simulink model "nl_model"  (R2021b)
settings: Solver=FixedStepAuto  StartTime=0.0  StopTime=10  FixedStep=0.01  MaxStep=0.01  RelTol=1e-3
values from neighbouring files (symbols this model uses):
  circ1 = monza    [sim_data.m]
  contact_treshold = 1e2    (= 100)    [sim_data.m]
  d = 0.021    [sim_data.m]
  H_cornice = 0.005    [sim_data.m]
  ICm = [IC(2), IC(4)]    [conversion_data.m]
  Kbbx = (mb * g * rb^2 * rm) / ((mb * rb^2 + Jb) * Ly)    (= 0.952057453416)    [sim_data.m]
  Kbby = (mb * g * rb^2 * rm) / ((mb * rb^2 + Jb) * Lx)    (= 1.22502497502)    [sim_data.m]
  lm = 0.072    [sim_data.m]
  Lx = 0.143    [sim_data.m]
  Lx_cornice = 0.15    [sim_data.m]
  Lx_plane = 0.15    [sim_data.m]
  Ly = 0.184    [sim_data.m]
  Ly_cornice = 0.20    (= 0.2)    [sim_data.m]
  Ly_plane = 0.20    (= 0.2)    [sim_data.m]
  Mot_Osci_Rang = [-90 ,90]    [sim_data.m]
  pt = 0.005    [sim_data.m]
  rb = 0.02    [sim_data.m]
  rm = 0.025    [sim_data.m]
  W_cornice = 0.05    [sim_data.m]
undefined symbols (not defined in the file or in its folder): DiscIntNeverNeededParam, h, Kx, Kxi, Ky, Kyi, slow, X, Y, Z
libraries: sm_lib x75, nesl_utility x9, simulink x7, dspstat3 x5, sharedschedule x3, slpidlib x2, dspsigops x1
(part 1 of 3)
settings Model: Creator=ernesto  LastModifiedBy=ernesto

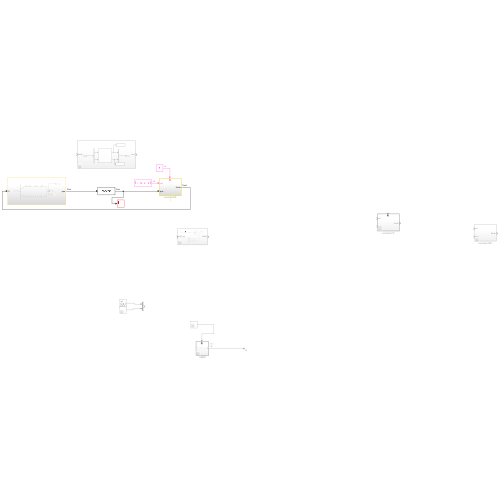
[thumbnail: Simulink's stored preview of the top-level diagram]
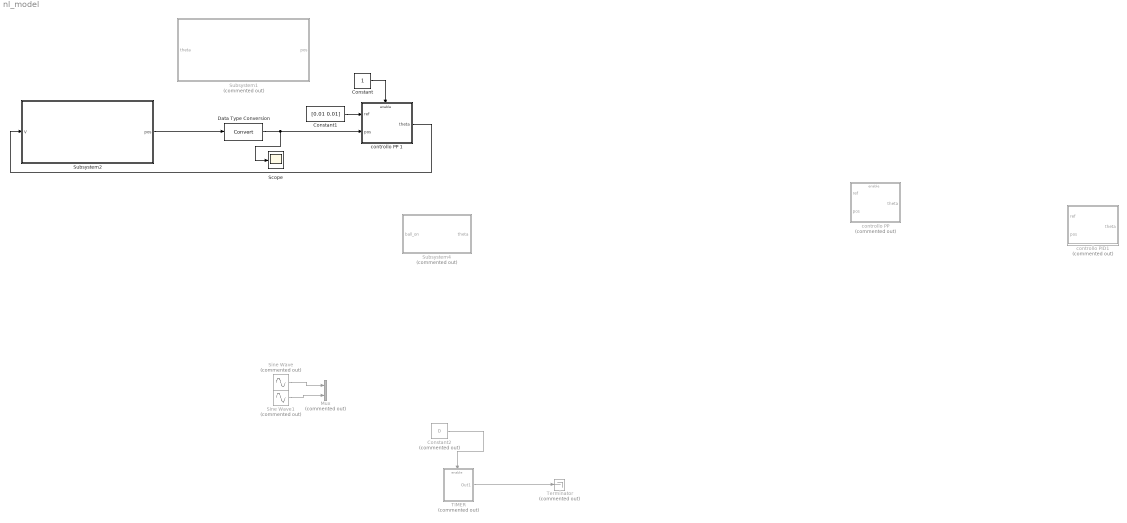
== system nl_model ==
  Constant : Constant
  Constant1 : Constant  Value=[0.01 0.01]
  Constant2 : Constant  Commented=on  Value=0  SampleTime=0.01
  Data Type Conversion : DataTypeConversion
  Mux : Mux  Commented=on  Inputs=2
  Scope : Scope
  Sine Wave : Sin  Commented=on  Amplitude=0.05  Frequency=2*pi*0.5  SampleTime=0.01
  Sine Wave1 : Sin  Commented=on  Amplitude=0.05  Frequency=2*pi*0.5  Phase=pi/2  SampleTime=0.01
  Subsystem1 : Subsystem  Commented=on
  Subsystem2 : Subsystem
  Subsystem4 : Subsystem  Commented=on
  TIMER : Subsystem  Commented=on  TreatAsAtomicUnit=on
  Terminator : Terminator  Commented=on
  controllo PID1 : Subsystem  Commented=on  SystemSampleTime=0.01
  "controllo PP " : Subsystem  Commented=on  SystemSampleTime=0.01
  controllo PP 1 : Subsystem  SystemSampleTime=0.01
  wires:
  Data Type Conversion/1 -> Scope/1, controllo PP 1/2("pos ")
  Constant2/1 -> TIMER/Enable
  TIMER/1(Out1) -> Terminator/1
  Sine Wave1/1 -> Mux/2
  Sine Wave/1 -> Mux/1
  Subsystem2/1(pos) -> Data Type Conversion/1
  controllo PP 1/1(theta) -> Subsystem2/1(V)
  Constant/1 -> controllo PP 1/Enable
  Constant1/1 -> controllo PP 1/1("ref ")

== system nl_model/Subsystem1 ==
  theta : Inport
  Demux : Demux  Outputs=2
  Mux : Mux  Inputs=2
  Subsystem : Subsystem
  To Workspace : ToWorkspace  VariableName=x  SaveFormat=Timeseries  SampleTime=-1
  To Workspace1 : ToWorkspace  VariableName=y  SaveFormat=Timeseries  SampleTime=-1
  pos : Outport
  wires:
  Subsystem/1(X_ideal) -> To Workspace/1, Mux/1  "position [m]"
  Subsystem/2(Y_ideal) -> To Workspace1/1, Mux/2  "position y [m]"
  Mux/1 -> pos/1
  Demux/2 -> Subsystem/2(ThetaY)
  Demux/1 -> Subsystem/1(ThetaX)
  theta/1 -> Demux/1

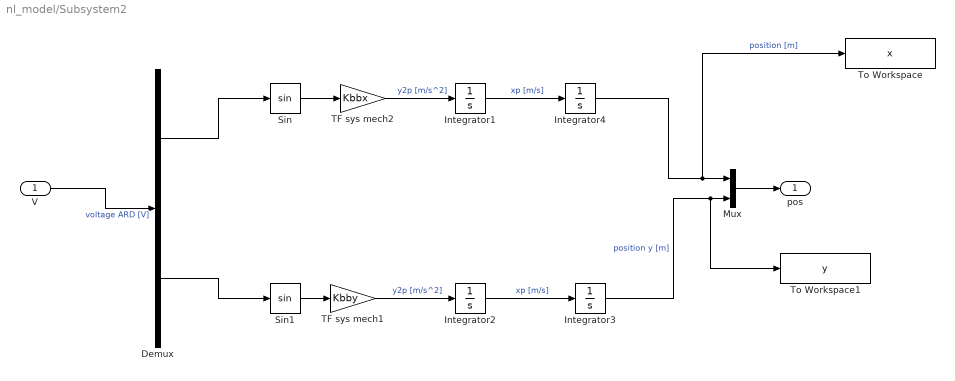
== system nl_model/Subsystem2 ==
  V : Inport
  Demux : Demux  Outputs=2
  Integrator{1..4} (4 alike) : Integrator
  Mux : Mux  Inputs=2
  Sin : Trigonometry
  Sin1 : Trigonometry
  TF sys mech1 : Gain  Gain=Kbby
  TF sys mech2 : Gain  Gain=Kbbx
  To Workspace : ToWorkspace  VariableName=x  SaveFormat=Timeseries  SampleTime=-1
  To Workspace1 : ToWorkspace  VariableName=y  SaveFormat=Timeseries  SampleTime=-1
  pos : Outport
  wires:
  Integrator3/1 -> To Workspace1/1, Mux/2  "position y [m]"
  V/1 -> Demux/1  "voltage ARD [V]"
  Mux/1 -> pos/1
  Integrator2/1 -> Integrator3/1  "xp [m/s]"
  TF sys mech1/1 -> Integrator2/1  "y2p [m/s^2]"
  Integrator1/1 -> Integrator4/1  "xp [m/s]"
  TF sys mech2/1 -> Integrator1/1  "y2p [m/s^2]"
  Sin/1 -> TF sys mech2/1
  Sin1/1 -> TF sys mech1/1
  Demux/2 -> Sin1/1
  Demux/1 -> Sin/1
  Integrator4/1 -> To Workspace/1, Mux/1  "position [m]"

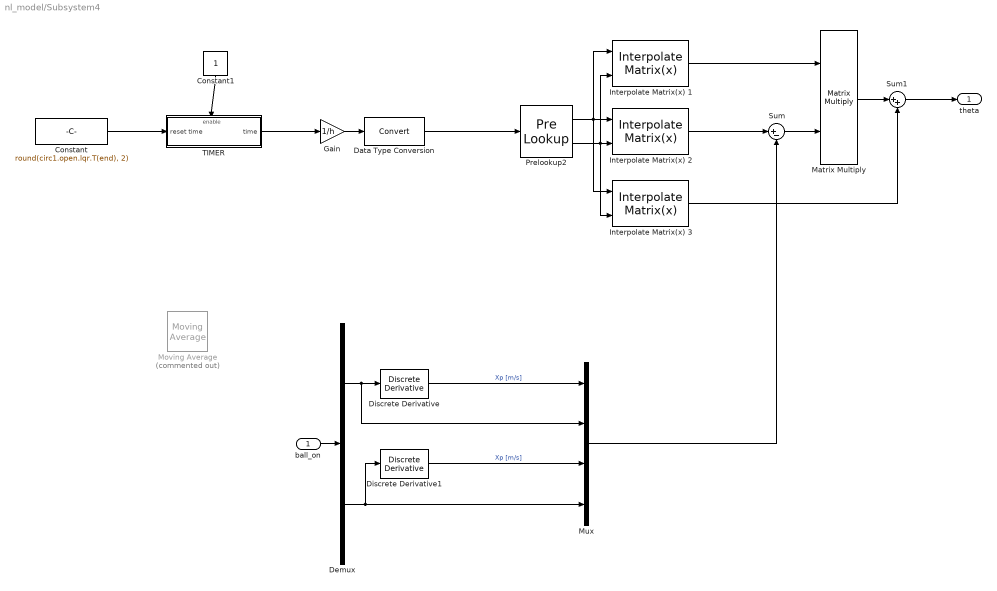
== system nl_model/Subsystem4 ==
  ball_on : Inport
  Constant : Constant  Value=round(circ1.open.lqr.T(end), 2)
  Constant1 : Constant
  Data Type Conversion : DataTypeConversion
  Demux : Demux  Outputs=2
  Discrete Derivative : simulink/Discrete/Discrete Derivative  gainval=1.0  ICPrevScaledInput=0.0  OutMin=[]  OutMax=[]  OutDataType=fixdt(1, 16)  OutScaling=2^-10  DoSatur=off
  Discrete Derivative1 : simulink/Discrete/Discrete Derivative  gainval=1.0  ICPrevScaledInput=0.0  OutMin=[]  OutMax=[]  OutDataType=fixdt(1, 16)  OutScaling=2^-10  DoSatur=off
  Gain : Gain  Gain=1/h
  Interpolate Matrix(x) 1 : sharedschedule/Interpolate Matrix(x)   matrix=circ1.open.lqr.K  aMode=aMode
      settings: SourceProductBaseCode=AE,PW,DR,MT,UV,VE
  Interpolate Matrix(x) 2 : sharedschedule/Interpolate Matrix(x)   matrix=circ1.open.lqr.xk  aMode=aMode
      settings: SourceProductBaseCode=AE,PW,DR,MT,UV,VE
  Interpolate Matrix(x) 3 : sharedschedule/Interpolate Matrix(x)   matrix=circ1.open.lqr.uk  aMode=aMode
      settings: SourceProductBaseCode=AE,PW,DR,MT,UV,VE
  Matrix Multiply : Product  Multiplication=Matrix(*)
  Moving Average : dspstat3/Moving Average  Commented=on  Method=Sliding window  ForgettingFactorPort=off  SpecifyWindowLength=on  WindowLength=20  ForgettingFactor=0.9  SimulateUsing=Code generation
  Mux : Mux
  Prelookup2 : PreLookup  BreakpointsData=([1:circ1.open.lqr.N])  IndexSearchMethod=Linear search  RemoveProtectionInput=on  BreakpointDataTypeStr=double  FractionDataTypeStr=double
  Sum : Sum  Inputs=|+-
  Sum1 : Sum  Inputs=|++
  TIMER : Subsystem  TreatAsAtomicUnit=on
  theta : Outport
  wires:
  ball_on/1 -> Demux/1
  Demux/1 -> Mux/2, Discrete Derivative/1
  Demux/2 -> Discrete Derivative1/1, Mux/4
  Discrete Derivative/1 -> Mux/1  "Xp [m/s]"
  Discrete Derivative1/1 -> Mux/3  "Xp [m/s]"
  Data Type Conversion/1 -> Prelookup2/1
  Interpolate Matrix(x) 1/1 -> Matrix Multiply/1
  Gain/1 -> Data Type Conversion/1
  Prelookup2/1 -> Interpolate Matrix(x) 1/1, Interpolate Matrix(x) 3/1, Interpolate Matrix(x) 2/1
  Prelookup2/2 -> Interpolate Matrix(x) 3/2, Interpolate Matrix(x) 1/2, Interpolate Matrix(x) 2/2
  Interpolate Matrix(x) 3/1 -> Sum1/2
  Interpolate Matrix(x) 2/1 -> Sum/1
  Sum/1 -> Matrix Multiply/2
  Sum1/1 -> theta/1
  Constant/1 -> TIMER/1(reset time)
  Mux/1 -> Sum/2
  Matrix Multiply/1 -> Sum1/1
  TIMER/1(time) -> Gain/1
  Constant1/1 -> TIMER/Enable

== system nl_model/TIMER ==
  Enable : EnablePort  StatesWhenEnabling=reset  ShowOutputPort=on
  Constant : Constant  SampleTime=-1
  Discrete-Time Integrator : DiscreteIntegrator  ExternalReset=either  SampleTime=-1  ICPrevOutput=DiscIntNeverNeededParam  ICPrevScaledInput=DiscIntNeverNeededParam
  Out1 : Outport
  wires:
  Constant/1 -> Discrete-Time Integrator/1
  Discrete-Time Integrator/1 -> Out1/1
  Enable/1 -> Discrete-Time Integrator/2

== system nl_model/controllo PID1 ==
  "ref " : Inport
  "pos " : Inport  Port=2
  Demux : Demux  Outputs=2
  Demux1 : Demux  Outputs=2
  Gain : Gain  Gain=-0.16
  Gain1 : Gain  Gain=-0.16
  Mux : Mux  Inputs=2
  PID Controller1 : slpidlib/PID Controller  Controller=PID  Form=Parallel  TimeDomain=Discrete-time  UseExternalTs=off  SampleTime=0.01  IntegratorMethod=Forward Euler  FilterMethod=Forward Euler  ControllerParametersSource=internal  P=22.5  I=0.2  D=18  UseFilter=on  N=20  TunerSelectOption=Transfer Function Based (PID Tuner App)  InitialConditionSource=internal  InitialConditionForIntegrator=0  InitialConditionForFilter=0  DifferentiatorICPrevScaledInput=0  ExternalReset=none  TrackingMode=off  Kt=1  LimitOutput=off  SatLimitsSource=internal  UpperSaturationLimit=inf  LowerSaturationLimit=-inf  LinearizeAsGain=on  AntiWindupMode=none  Kb=1  POutMin=[]  POutMax=[]  IOutMin=[]  IOutMax=[]  DOutMin=[]  DOutMax=[]  NOutMin=[]  NOutMax=[]  SumOutMin=[]  SumOutMax=[]  SaturationOutMin=[]  SaturationOutMax=[]  PParamMin=[]  PParamMax=[]  IParamMin=[]  IParamMax=[]  DParamMin=[]  DParamMax=[]  NParamMin=[]  NParamMax=[]  KbParamMin=[]  KbParamMax=[]  KtParamMin=[]  KtParamMax=[]  KbOutMin=[]  KbOutMax=[]  KtOutMin=[]  KtOutMax=[]  IntegratorOutMin=[]  IntegratorOutMax=[]  FilterOutMin=[]  FilterOutMax=[]  SumI1OutMin=[]  SumI1OutMax=[]  SumI2OutMin=[]  SumI2OutMax=[]  SumI3OutMin=[]  SumI3OutMax=[]  SumI4OutMin=[]  SumI4OutMax=[]  SumDOutMin=[]  SumDOutMax=[]  DifferentiatorOutMin=[]  DifferentiatorOutMax=[]  FilterDiffOutCoefMin=[]  FilterDiffOutCoefMax=[]  ReciprocalOutMin=[]  ReciprocalOutMax=[]  SumDenOutMin=[]  SumDenOutMax=[]  SumNumOutMin=[]  SumNumOutMax=[]  DivideOutMin=[]  DivideOutMax=[]  UdiffTsProdOutMin=[]  UdiffTsProdOutMax=[]  NTsProdOutMin=[]  NTsProdOutMax=[]  UintegralTsProdOutMin=[]  UintegralTsProdOutMax=[]  UngainTsProdOutMin=[]  UngainTsProdOutMax=[]  IntegratorContinuousStateAttributes=''  IntegratorStateMustResolveToSignalObject=off  IntegratorRTWStateStorageClass=Auto  FilterContinuousStateAttributes=''  FilterStateMustResolveToSignalObject=off  FilterRTWStateStorageClass=Auto  ParallelPVariant=InternalParameters  IdealPVariant=Disabled  IVariant=InternalParameters  DVariant=InternalParameters  IntegratorVariant=Discrete  SatVariant=Disabled  AWVariant=Passthrough  PCopyVariant=Disabled  TRVariant=Disabled  FdbkBlocksVariant=Forward  IdealPFdbkVariant=Disabled  SatFdbkVariant=Disabled  DerivativeFilterVariant=ForwardEulerFilter  NVariant=InternalParameters  NCopyVariant=Disabled  FilterICVariant=InternalICsFilter  IntegratorICVariant=InternalICs  ExternalResetVariant=Disabled  TRSumVariant=Passthrough  SumFdbkVariant=Disabled  SumVariant=Sum_PID  TsampFilterVariant=InternalTs  TsampNgainVariant=Passthrough  TsampIntegralVariant=Passthrough  ExternalSaturationOutDataTypeStr=Inherit: Same as second input
  PID Controller4 : slpidlib/PID Controller  Controller=PID  Form=Parallel  TimeDomain=Discrete-time  UseExternalTs=off  SampleTime=0.01  IntegratorMethod=Forward Euler  FilterMethod=Forward Euler  ControllerParametersSource=internal  P=22.5  I=0.2  D=18  UseFilter=on  N=20  TunerSelectOption=Transfer Function Based (PID Tuner App)  InitialConditionSource=internal  InitialConditionForIntegrator=0  InitialConditionForFilter=0  DifferentiatorICPrevScaledInput=0  ExternalReset=none  TrackingMode=off  Kt=1  LimitOutput=off  SatLimitsSource=internal  UpperSaturationLimit=inf  LowerSaturationLimit=-inf  LinearizeAsGain=on  AntiWindupMode=none  Kb=1  POutMin=[]  POutMax=[]  IOutMin=[]  IOutMax=[]  DOutMin=[]  DOutMax=[]  NOutMin=[]  NOutMax=[]  SumOutMin=[]  SumOutMax=[]  SaturationOutMin=[]  SaturationOutMax=[]  PParamMin=[]  PParamMax=[]  IParamMin=[]  IParamMax=[]  DParamMin=[]  DParamMax=[]  NParamMin=[]  NParamMax=[]  KbParamMin=[]  KbParamMax=[]  KtParamMin=[]  KtParamMax=[]  KbOutMin=[]  KbOutMax=[]  KtOutMin=[]  KtOutMax=[]  IntegratorOutMin=[]  IntegratorOutMax=[]  FilterOutMin=[]  FilterOutMax=[]  SumI1OutMin=[]  SumI1OutMax=[]  SumI2OutMin=[]  SumI2OutMax=[]  SumI3OutMin=[]  SumI3OutMax=[]  SumI4OutMin=[]  SumI4OutMax=[]  SumDOutMin=[]  SumDOutMax=[]  DifferentiatorOutMin=[]  DifferentiatorOutMax=[]  FilterDiffOutCoefMin=[]  FilterDiffOutCoefMax=[]  ReciprocalOutMin=[]  ReciprocalOutMax=[]  SumDenOutMin=[]  SumDenOutMax=[]  SumNumOutMin=[]  SumNumOutMax=[]  DivideOutMin=[]  DivideOutMax=[]  UdiffTsProdOutMin=[]  UdiffTsProdOutMax=[]  NTsProdOutMin=[]  NTsProdOutMax=[]  UintegralTsProdOutMin=[]  UintegralTsProdOutMax=[]  UngainTsProdOutMin=[]  UngainTsProdOutMax=[]  IntegratorContinuousStateAttributes=''  IntegratorStateMustResolveToSignalObject=off  IntegratorRTWStateStorageClass=Auto  FilterContinuousStateAttributes=''  FilterStateMustResolveToSignalObject=off  FilterRTWStateStorageClass=Auto  ParallelPVariant=InternalParameters  IdealPVariant=Disabled  IVariant=InternalParameters  DVariant=InternalParameters  IntegratorVariant=Discrete  SatVariant=Disabled  AWVariant=Passthrough  PCopyVariant=Disabled  TRVariant=Disabled  FdbkBlocksVariant=Forward  IdealPFdbkVariant=Disabled  SatFdbkVariant=Disabled  DerivativeFilterVariant=ForwardEulerFilter  NVariant=InternalParameters  NCopyVariant=Disabled  FilterICVariant=InternalICsFilter  IntegratorICVariant=InternalICs  ExternalResetVariant=Disabled  TRSumVariant=Passthrough  SumFdbkVariant=Disabled  SumVariant=Sum_PID  TsampFilterVariant=InternalTs  TsampNgainVariant=Passthrough  TsampIntegralVariant=Passthrough  ExternalSaturationOutDataTypeStr=Inherit: Same as second input
  Sum2 : Sum  Inputs=|-+
  Sum3 : Sum  Inputs=|-+
  theta : Outport
  wires:
  "ref "/1 -> Demux1/1
  "pos "/1 -> Demux/1
  Mux/1 -> theta/1
  Demux/1 -> Sum2/1
  Demux/2 -> Sum3/1
  Demux1/1 -> Sum2/2
  Demux1/2 -> Sum3/2
  Sum3/1 -> PID Controller1/1
  PID Controller1/1 -> Gain1/1
  Sum2/1 -> PID Controller4/1
  PID Controller4/1 -> Gain/1
  Gain/1 -> Mux/1
  Gain1/1 -> Mux/2

== system nl_model/controllo PP  ==
  "ref " : Inport
  "pos " : Inport  Port=2
  Enable : EnablePort  StatesWhenEnabling=reset  ShowOutputPort=on
  Demux : Demux  Outputs=2
  Demux1 : Demux  Outputs=2
  Mux : Mux  Inputs=2
  PPX 1 : Subsystem
  PPX 2 : Subsystem
  Sum2 : Sum  Inputs=|-+
  Sum3 : Sum  Inputs=|-+
  theta : Outport
  wires:
  "ref "/1 -> Demux1/1
  "pos "/1 -> Demux/1
  Demux/1 -> PPX 1/1("pos "), Sum2/1
  Demux/2 -> PPX 2/1("pos "), Sum3/1
  Demux1/1 -> Sum2/2
  Demux1/2 -> Sum3/2
  Sum3/1 -> PPX 2/2(err)
  Sum2/1 -> PPX 1/2(err)
  PPX 2/1(V) -> Mux/2
  PPX 1/1(V) -> Mux/1
  Mux/1 -> theta/1
  Enable/1 -> PPX 2/3(tr), PPX 1/3(tr)

== system nl_model/controllo PP 1 ==
  "ref " : Inport
  "pos " : Inport  Port=2
  Enable : EnablePort  StatesWhenEnabling=reset  ShowOutputPort=on
  Demux : Demux  Outputs=2
  Demux1 : Demux  Outputs=2
  Mux : Mux  Inputs=2
  PPX 1 : Subsystem
  PPX 2 : Subsystem
  Sum2 : Sum  Inputs=|-+
  Sum3 : Sum  Inputs=|-+
  theta : Outport
  wires:
  "ref "/1 -> Demux1/1
  "pos "/1 -> Demux/1
  Demux/1 -> PPX 1/1("pos "), Sum2/1
  Demux/2 -> PPX 2/1("pos "), Sum3/1
  Demux1/1 -> Sum2/2
  Demux1/2 -> Sum3/2
  Sum3/1 -> PPX 2/2(err)
  Sum2/1 -> PPX 1/2(err)
  PPX 2/1(V) -> Mux/2
  PPX 1/1(V) -> Mux/1
  Mux/1 -> theta/1
  Enable/1 -> PPX 2/3(tr), PPX 1/3(tr)

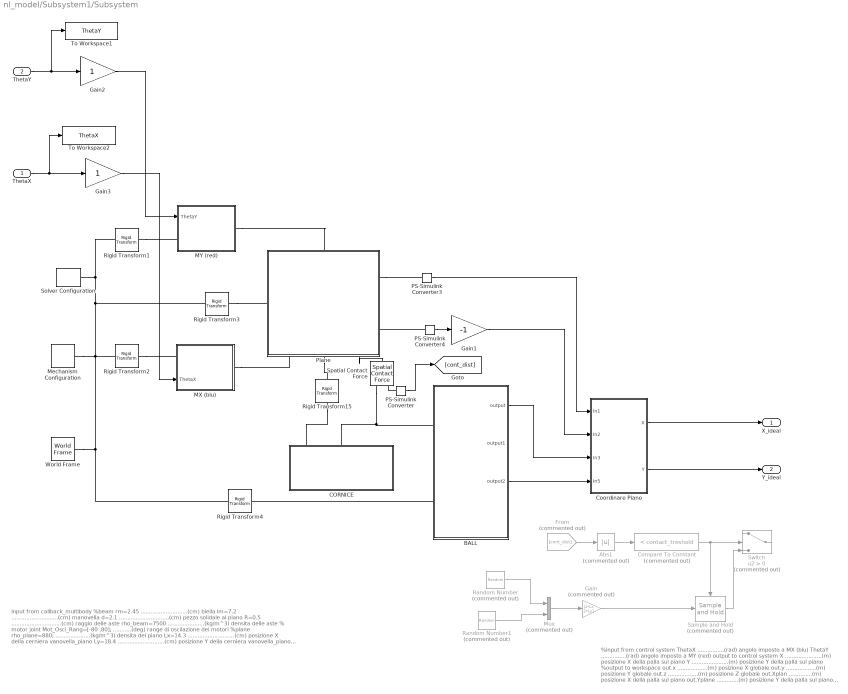
== system nl_model/Subsystem1/Subsystem ==
  note: %input from control system
      | ThetaX ................(rad) angolo imposto a MX (blu)
      | ThetaY ...............(rad) angolo imposto a MY (red)
      |
      | output to control system
      | X ......................(m) posizione X della palla sul piano
      | Y ......................(m) posizione Y della palla sul piano
      |
      | %output to workspace
      | out.x ..................(m) posizione X globale
      | out.y ..................(m) posizione Y globale
      | out.z ..................(m) posizione Z globale
      | out.Xplan ..............(m) posizione X della palla sul piano
      | out.Yplane .............(m) posizione Y della palla sul piano
      | out.angX ...............(rad) angolo di rotazione intorno a Y
      | out.angZ ...............(rad) angolo di rotazione intorno a X
  note: input from callback_multibody
      | %beam
      | rm=2.45 ............................(cm) biella
      | lm=7.2 ............................(cm) manovella
      | d=2.1 ..............................(cm) pezzo solidale al piano
      | R=0.5 ..............................(cm) raggio delle aste
      | rho_beam=7500 ......................(kg/m^3) densita delle aste
      | % motor joint
      | Mot_Osci_Rang=[-80 ,80]; ...........(deg) range di oscilazione dei motori
      | %plane
      | rho_plane=880; .....................(kg/m^3) densita del piano
      | Lx=14.3 ............................(cm) posizione X della cerniera vanovella_piano
      | Ly=18.4 ............................(cm) posizione Y della cerniera vanovella_piano
      | Lx_plane=15 ........................(cm) dimensione X piano (met della lunghezza)
      | Ly_plane=20 ........................(cm) dimensione Y piano (met della lunghezza)
      | %ball
      | rho_ball=8000 ......................(kg/m^3) densita della sfera
      | R_ball=2 ...........................(cm) raggio della sfera
      | X_start=0 ..........................(cm) posizione X di partenza della palla
      | Y_start=0 ..........................(cm) posizione Y di partenza della palla
      | Z_start=0 ..........................(cm) posizione X di partenza della palla (Z=0 palla e piano in contatto)
      | %cornice
      | Lx_cornice=15 ......................(cm) dimensione X della cornice (meta)
      | Ly_cornice=20 ......................(cm) dimensione Y della cornice (meta)
      | H_cornice=0.5 ......................(cm) spessore cornice
      | W_cornice=2 ........................(cm) altezza cornice
  ThetaX : Inport
  ThetaY : Inport  Port=2
  Abs1 : Abs  Commented=on
  BALL : Subsystem
  CORNICE : Subsystem
  Compare To Constant : simulink/Logic and Bit Operations/Compare To Constant  Commented=on  relop=<  const=contact_treshold  OutDataTypeStr=boolean
  Coordinare Piano : Subsystem
  From : From  Commented=on  GotoTag=cont_dist
  Gain : Gain  Commented=on  Gain=[2*Lx 2*Ly]
  Gain1 : Gain  Gain=-1
  Gain2 : Gain
  Gain3 : Gain
  MX (blu) : Subsystem
      settings: PortSchema="{\"entries\":[{\"content\":{\"sides\":[{\"content\":{\"connectorIds\":[\"LConn1\",\"In1\"]},\"type\":\"ConnectorPlacement.EquallySpacedRectSide\",\"uuid\":\"f8f12517-1207-4299-855f-f75f42ab5f4f\"},{\"content\":{\"connectorIds\":[\"RConn1\"],\"side\":\"RIGHT\"},\"type\":\"ConnectorPlacement.EquallySpacedRectSide\",\"uuid\":\"0d1367b1-3b15-4c68-a856-5ade25dab0e5\"},{\"content\":{\"connectorIds\":[],\"side\":\"TOP\"},\"type\":\"ConnectorPlacement.EquallySpacedRectSide\",\"uuid\":\"8b5913a7-4fd7-423b-8085-c56b4a024020\"}]},\"type\":\"ConnectorPlacement.EquallySpacedConnector\",\"uuid\":\"558f39aa-b3e3-4037-8179-13dbf31ad577\"}],\"packageUris\":[\"http://schema.mathworks.com/mf0/Connector/R2020b\"],\"version\":\"1.0\"}"
  MY (red) : Subsystem
  Mechanism Configuration : sm_lib/Utilities/Mechanism Configuration  UniformGravity=Constant  GravityVector=[0 -9.80665 0]  GravityUnits=m/s^2  LinearizationDelta=0.001  JointModeTransitionNonlinearIterations=2
  Mux : Mux  Commented=on  Inputs=2
  PS-Simulink Converter : nesl_utility/PS-Simulink Converter  PhysicalDomain=network_engine_domain  SubClassName=ps_output  LeftPortType=input  RightPortType=output  PseudoPeriodic=off  Frequencies=[]  Unit=inherit  AffineConversion=off
      settings: SourceProductBaseCode=PW,SS
  PS-Simulink Converter3 : nesl_utility/PS-Simulink Converter  PhysicalDomain=network_engine_domain  SubClassName=ps_output  LeftPortType=input  RightPortType=output  PseudoPeriodic=off  Frequencies=[]  Unit=inherit  AffineConversion=off
      settings: SourceProductBaseCode=PW,SS
  PS-Simulink Converter4 : nesl_utility/PS-Simulink Converter  PhysicalDomain=network_engine_domain  SubClassName=ps_output  LeftPortType=input  RightPortType=output  PseudoPeriodic=off  Frequencies=[]  Unit=inherit  AffineConversion=off
      settings: SourceProductBaseCode=PW,SS
  Plane : Subsystem
      settings: PortSchema="{\"entries\":[{\"content\":{\"sides\":[{\"content\":{\"connectorIds\":[\"LConn1\"]},\"type\":\"ConnectorPlacement.EquallySpacedRectSide\",\"uuid\":\"fb1680d6-c609-4aca-a7f0-b5f55d3f0aaf\"},{\"content\":{\"connectorIds\":[\"RConn1\",\"RConn2\"],\"side\":\"RIGHT\"},\"type\":\"ConnectorPlacement.EquallySpacedRectSide\",\"uuid\":\"63411687-c407-4582-b1a6-cafd628fb3b5\"},{\"content\":{\"connectorIds\":[\"LConn2\"],\"side\":\"TOP\"},\"type\":\"ConnectorPlacement.EquallySpacedRectSide\",\"uuid\":\"ba6745b0-0d49-4eb1-9c08-15e05c1cd980\"},{\"content\":{\"connectorIds\":[\"RConn3\",\"RConn4\",\"RConn5\"],\"side\":\"BOTTOM\"},\"type\":\"ConnectorPlacement.EquallySpacedRectSide\",\"uuid\":\"c7cb78ef-fa1b-4f0d-9ee3-e2765f49442b\"}]},\"type\":\"ConnectorPlacement.EquallySpacedConnector\",\"uuid\":\"606e2972-e222-401b-95ff-46f36b1a383d\"}],\"packageUris\":[\"http://schema.mathworks.com/mf0/Connector/R2020b\"],\"version\":\"1.0\"}"
  Random Number : RandomNumber  Commented=on  SampleTime=0.01
  Random Number1 : RandomNumber  Commented=on  SampleTime=0.01
  Rigid Transform1 : sm_lib/Frames and Transforms/Rigid Transform  TranslationMethod=Cartesian  TranslationStandardOffset=0  TranslationLengthUnit=m  TranslationStandardAxis=+Z  TranslationCartesianOffset=[-Lx -lm-d rm]  TranslationROffset=0  TranslationROffsetUnits=m  TranslationZOffset=0  TranslationZOffsetUnits=m  TranslationThetaOffset=0  TranslationThetaOffsetUnits=deg  RotationMethod=RotationSequence  RotationAngleUnits=deg  RotationStandardAxis=+Z  RotationAngle=0.0  RotationArbitraryAxis=[0 0 1]  FollAlignAxisA=+X  BaseAlignAxisA=+Y  FollAlignAxisB=+Y  BaseAlignAxisB=+Z  RotationSequenceAxes=FollowerAxes  RotationSequence=XYZ  RotationSequenceAngles=[0 90 0]  RotationSequenceAnglesUnits=deg  RotationMatrix=[1 0 0; 0 1 0; 0 0 1]
  Rigid Transform15 : sm_lib/Frames and Transforms/Rigid Transform  TranslationMethod=Cartesian  TranslationStandardOffset=0  TranslationLengthUnit=m  TranslationStandardAxis=+Z  TranslationCartesianOffset=[0 0 0]  TranslationROffset=0  TranslationROffsetUnits=m  TranslationZOffset=0  TranslationZOffsetUnits=m  TranslationThetaOffset=0  TranslationThetaOffsetUnits=deg  RotationMethod=RotationSequence  RotationAngleUnits=deg  RotationStandardAxis=+Z  RotationAngle=0.0  RotationArbitraryAxis=[0 0 1]  FollAlignAxisA=+X  BaseAlignAxisA=+Y  FollAlignAxisB=+Y  BaseAlignAxisB=+Z  RotationSequenceAxes=FollowerAxes  RotationSequence=XYZ  RotationSequenceAngles=[0 0 0]  RotationSequenceAnglesUnits=deg  RotationMatrix=[1 0 0; 0 1 0; 0 0 1]
  Rigid Transform2 : sm_lib/Frames and Transforms/Rigid Transform  TranslationMethod=Cartesian  TranslationStandardOffset=0  TranslationLengthUnit=m  TranslationStandardAxis=+Z  TranslationCartesianOffset=[rm -lm-d -Ly]  TranslationROffset=0  TranslationROffsetUnits=m  TranslationZOffset=0  TranslationZOffsetUnits=m  TranslationThetaOffset=0  TranslationThetaOffsetUnits=deg  RotationMethod=RotationSequence  RotationAngleUnits=deg  RotationStandardAxis=+Z  RotationAngle=0.0  RotationArbitraryAxis=[0 0 1]  FollAlignAxisA=+X  BaseAlignAxisA=+Y  FollAlignAxisB=+Y  BaseAlignAxisB=+Z  RotationSequenceAxes=FollowerAxes  RotationSequence=XYZ  RotationSequenceAngles=[0 180 0]  RotationSequenceAnglesUnits=deg  RotationMatrix=[1 0 0; 0 1 0; 0 0 1]
  Rigid Transform3 : sm_lib/Frames and Transforms/Rigid Transform  TranslationMethod=Cartesian  TranslationStandardOffset=0  TranslationLengthUnit=m  TranslationStandardAxis=+Z  TranslationCartesianOffset=[0 -pt/2 0]  TranslationROffset=0  TranslationROffsetUnits=m  TranslationZOffset=0  TranslationZOffsetUnits=m  TranslationThetaOffset=0  TranslationThetaOffsetUnits=deg  RotationMethod=RotationSequence  RotationAngleUnits=deg  RotationStandardAxis=+Z  RotationAngle=0.0  RotationArbitraryAxis=[0 0 1]  FollAlignAxisA=+X  BaseAlignAxisA=+Y  FollAlignAxisB=+Y  BaseAlignAxisB=+Z  RotationSequenceAxes=FollowerAxes  RotationSequence=XYZ  RotationSequenceAngles=[90 0 0]  RotationSequenceAnglesUnits=deg  RotationMatrix=[1 0 0; 0 1 0; 0 0 1]
  Rigid Transform4 : sm_lib/Frames and Transforms/Rigid Transform  TranslationMethod=Cartesian  TranslationStandardOffset=0  TranslationLengthUnit=m  TranslationStandardAxis=+Z  TranslationCartesianOffset="[ICm(2) rb  ICm(1)]"  TranslationROffset=0  TranslationROffsetUnits=m  TranslationZOffset=0  TranslationZOffsetUnits=m  TranslationThetaOffset=0  TranslationThetaOffsetUnits=deg  RotationMethod=RotationSequence  RotationAngleUnits=deg  RotationStandardAxis=+Z  RotationAngle=0.0  RotationArbitraryAxis=[0 0 1]  FollAlignAxisA=+X  BaseAlignAxisA=+Y  FollAlignAxisB=+Y  BaseAlignAxisB=+Z  RotationSequenceAxes=FollowerAxes  RotationSequence=XYZ  RotationSequenceAngles=[0 0 0]  RotationSequenceAnglesUnits=deg  RotationMatrix=[1 0 0; 0 1 0; 0 0 1]
  Sample and Hold : dspsigops/Sample and Hold  Commented=on  trig=Rising edge  initCond=0  latchinput=off
  Solver Configuration : nesl_utility/Solver Configuration  PhysicalDomain=network_engine_domain  SubClassName=solver  LeftPortType=input  RightPortType=generic  Tones=[]  Harmonics=[]  SimulateNoise=off  Profile=off  UseLocalSampling=off  EnableSwitchedLinearOptims=on  FrequencyDomain=off  UseCCode=off  RelTol=0.001  AbsTol=1e-06  MinStep=1e-09  ToWorkspace=off  RevertToSquareIcSolve=off  NumHomotopyIterations=100  PhasorMode=off  PhasorModeNumHarmonics=1  DoDC=off  ResidualTolerance=1e-09  UseLocalSolver=off  LocalSolverChoice=NE_BACKWARD_EULER_ADVANCER  LocalSolverSampleTime=0.001  DoFixedCost=off  MaxNonlinIter=3  MaxModeIter=2  ComputeImpulses=off  ImpulseIterations=2  LinearAlgebra=Sparse  EquationFormulation=NE_TIME_EF  DelaysMemoryBudget=1024  AutomaticFiltering=on  FilteringTimeConstant=0.001  PartitionStorageMethod=AS_NEEDED  PartitionMemoryBudget=1024  PartitionMethod=FAST
      settings: SourceProductBaseCode=PW,SS
  Spatial Contact Force : sm_lib/Forces and Torques/Spatial Contact Force  CoefficientOfDynamicFriction=mu_dynamic  CoefficientOfStaticFriction=mu_static  SenseContactBaseRotation=off  SenseContactBaseTranslation=off  NormalDamping=1e1  NormalDampingUnits=N/(m/s)  SenseContactFollowerRotation=off  SenseContactFollowerTranslation=off  SenseContactSignal=off  NormalStiffness=1e3  NormalStiffnessUnits=N/m  FrictionalCriticalVelocity=1e-3  FrictionalCriticalVelocityUnits=m/s  ZeroCrossDetectContactStartAndEnd=off  FrictionType=SmoothStickSlip  SenseFrictionalForceMagnitude=off  SenseNormalForceMagnitude=off  NormalForceType=SmoothSpringDamper  SenseNormalVelocity=off  SenseSeparationDistance=on  SenseTangentialVelocity=off  SenseTangentialVelocityMagnitude=off  NormalTransitionRegionWidth=5e-4  NormalTransitionRegionWidthUnits=m
  Switch : Switch  Commented=on  Criteria=u2 > Threshold
  To Workspace1 : ToWorkspace  VariableName=ThetaY  SaveFormat=Timeseries  SampleTime=-1
  To Workspace2 : ToWorkspace  VariableName=ThetaX  SaveFormat=Timeseries  SampleTime=-1
  World Frame : sm_lib/Frames and Transforms/World Frame
  X_ideal : Outport
  Y_ideal : Outport  Port=2
  wires:
  Gain3/1 -> MX (blu)/1(ThetaX)
  ThetaX/1 -> To Workspace2/1, Gain3/1
  ThetaY/1 -> Gain2/1, To Workspace1/1
  PS-Simulink Converter3/1 -> Coordinare Piano/1(In1)
  Gain2/1 -> MY (red)/1(ThetaY)
  PS-Simulink Converter4/1 -> Gain1/1
  Gain1/1 -> Coordinare Piano/2(In2)
  BALL/1(output) -> Coordinare Piano/3(In3)
  BALL/3(output2) -> Coordinare Piano/4(In5)
  PS-Simulink Converter/1 -> [cont_dist]
  From/1 -> Abs1/1
  Abs1/1 -> Compare To Constant/1
  Compare To Constant/1 -> Switch/2, Sample and Hold/Trigger
  Mux/1 -> Gain/1
  Sample and Hold/1 -> Switch/3
  Gain/1 -> Sample and Hold/1
  Random Number/1 -> Mux/1
  Random Number1/1 -> Mux/2
  Coordinare Piano/1(X) -> X_ideal/1
  Coordinare Piano/2(Y) -> Y_ideal/1
  connections:
  Mechanism Configuration/RConn1 -- Solver Configuration/RConn1 -- Rigid Transform1/LConn1 -- Rigid Transform3/LConn1 -- Rigid Transform2/LConn1 -- Rigid Transform4/LConn1 -- World Frame/RConn1
  Plane/RConn1 -- PS-Simulink Converter3/LConn1
  Rigid Transform3/RConn1 -- Plane/LConn1
  MY (red)/RConn1 -- Plane/LConn2
  MX (blu)/RConn1 -- Plane/RConn3
  Rigid Transform2/RConn1 -- MX (blu)/LConn1
  PS-Simulink Converter4/LConn1 -- Plane/RConn2
  Plane/RConn5 -- Spatial Contact Force/LConn1
  Plane/RConn4 -- Rigid Transform15/LConn1
  Rigid Transform15/RConn1 -- CORNICE/RConn1
  Rigid Transform1/RConn1 -- MY (red)/LConn1
  Spatial Contact Force/RConn1 -- BALL/LConn1 -- CORNICE/RConn2
  BALL/LConn2 -- Rigid Transform4/RConn1
  PS-Simulink Converter/LConn1 -- Spatial Contact Force/RConn2

== system nl_model/Subsystem4/TIMER ==
  reset time : Inport
  Enable : EnablePort  StatesWhenEnabling=reset  ShowOutputPort=on
  Constant : Constant  SampleTime=-1
  Delay1 : Delay  DelayLength=1  InitialCondition=0
  Discrete-Time Integrator : DiscreteIntegrator  ExternalReset=either  SampleTime=-1  ICPrevOutput=DiscIntNeverNeededParam  ICPrevScaledInput=DiscIntNeverNeededParam
  Logical Operator1 : Logic  AllPortsSameDT=off  OutDataTypeStr=boolean
  Relational Operator : RelationalOperator  OutDataTypeStr=boolean  RndMeth=Simplest
  time : Outport
  wires:
  Constant/1 -> Discrete-Time Integrator/1
  Discrete-Time Integrator/1 -> Delay1/1, time/1
  Logical Operator1/1 -> Discrete-Time Integrator/2
  Enable/1 -> Logical Operator1/1
  Relational Operator/1 -> Logical Operator1/2
  reset time/1 -> Relational Operator/2
  Delay1/1 -> Relational Operator/1

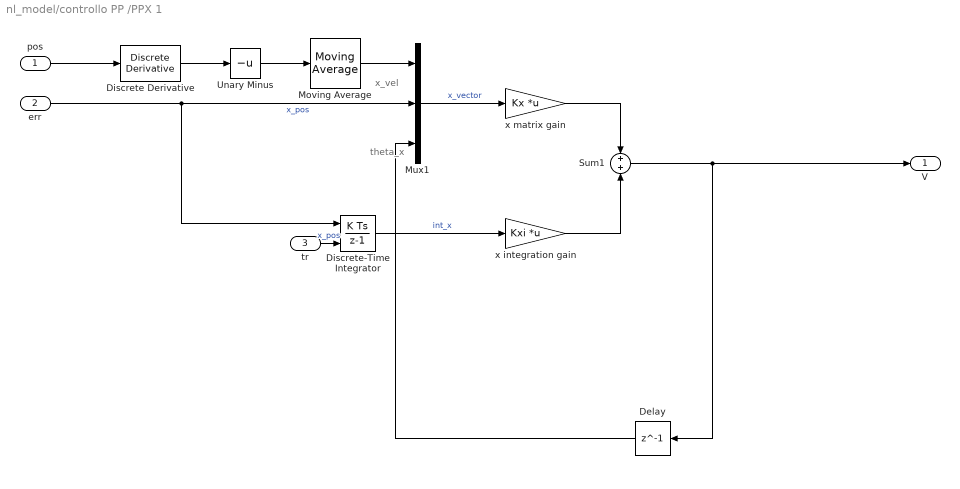
== system nl_model/controllo PP /PPX 1 ==
  note: theta_x
  note: x_vel
  "pos " : Inport
  err : Inport  Port=2
  tr : Inport  Port=3
  Delay : Delay  DelayLength=1  InitialCondition=0
  Discrete Derivative : simulink/Discrete/Discrete Derivative  gainval=1.0  ICPrevScaledInput=0.0  OutMin=[]  OutMax=[]  OutDataType=fixdt(1, 16)  OutScaling=2^-10  DoSatur=off
  Discrete-Time Integrator : DiscreteIntegrator  ExternalReset=rising  SampleTime=-1  ICPrevOutput=DiscIntNeverNeededParam  ICPrevScaledInput=DiscIntNeverNeededParam
  Moving Average : dspstat3/Moving Average  Method=Sliding window  ForgettingFactorPort=off  SpecifyWindowLength=on  WindowLength=20  ForgettingFactor=0.9  SimulateUsing=Code generation
  Mux1 : Mux  Inputs=3
  Sum1 : Sum  Inputs=+|+
  Unary Minus : UnaryMinus
  x integration gain : Gain  Gain=Kxi  Multiplication=Matrix(K*u)
  x matrix gain : Gain  Gain=Kx  Multiplication=Matrix(K*u)
  V : Outport
  wires:
  x matrix gain/1 -> Sum1/1
  Mux1/1 -> x matrix gain/1  "x_vector"
  x integration gain/1 -> Sum1/2
  err/1 -> Discrete-Time Integrator/1, Mux1/2  "x_pos"
  Discrete-Time Integrator/1 -> x integration gain/1  "int_x"
  "pos "/1 -> Discrete Derivative/1
  Delay/1 -> Mux1/3
  Sum1/1 -> Delay/1, V/1
  tr/1 -> Discrete-Time Integrator/2  "x_pos"
  Discrete Derivative/1 -> Unary Minus/1
  Unary Minus/1 -> Moving Average/1
  Moving Average/1 -> Mux1/1

== system nl_model/controllo PP /PPX 2 ==
  note: theta_x
  note: x_vel
  "pos " : Inport
  err : Inport  Port=2
  tr : Inport  Port=3
  Delay : Delay  DelayLength=1  InitialCondition=0
  Discrete Derivative : simulink/Discrete/Discrete Derivative  gainval=1.0  ICPrevScaledInput=0.0  OutMin=[]  OutMax=[]  OutDataType=fixdt(1, 16)  OutScaling=2^-10  DoSatur=off
  Discrete-Time Integrator : DiscreteIntegrator  ExternalReset=rising  SampleTime=-1  ICPrevOutput=DiscIntNeverNeededParam  ICPrevScaledInput=DiscIntNeverNeededParam
  Moving Average : dspstat3/Moving Average  Method=Sliding window  ForgettingFactorPort=off  SpecifyWindowLength=on  WindowLength=10  ForgettingFactor=0.9  SimulateUsing=Code generation
  Mux1 : Mux  Inputs=3
  Sum1 : Sum  Inputs=+|+
  x integration gain : Gain  Gain=Kyi  Multiplication=Matrix(K*u)
  x matrix gain : Gain  Gain=Ky  Multiplication=Matrix(K*u)
  V : Outport
  wires:
  x matrix gain/1 -> Sum1/1
  Mux1/1 -> x matrix gain/1  "x_vector"
  x integration gain/1 -> Sum1/2
  err/1 -> Discrete-Time Integrator/1, Mux1/2  "x_pos"
  Discrete-Time Integrator/1 -> x integration gain/1  "int_x"
  "pos "/1 -> Discrete Derivative/1
  Delay/1 -> Mux1/3
  Sum1/1 -> Delay/1, V/1
  tr/1 -> Discrete-Time Integrator/2  "x_pos"
  Discrete Derivative/1 -> Moving Average/1
  Moving Average/1 -> Mux1/1

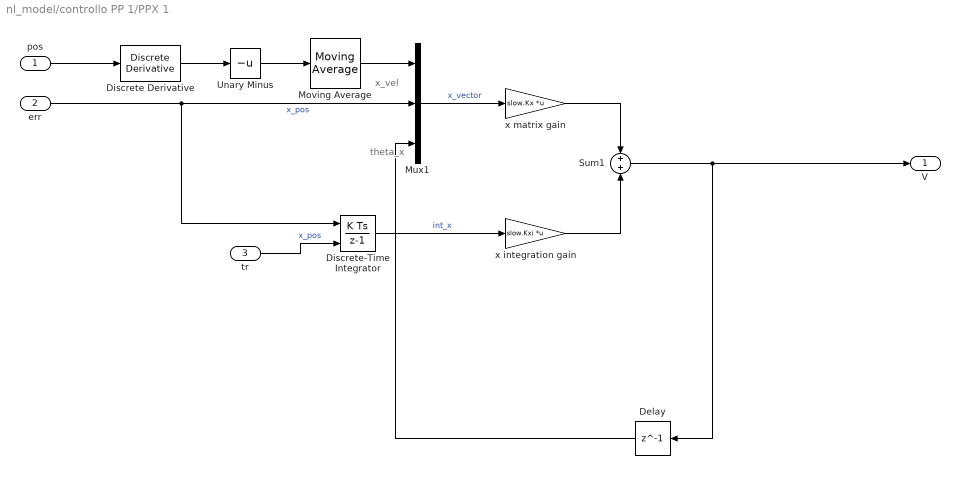
== system nl_model/controllo PP 1/PPX 1 ==
  note: theta_x
  note: x_vel
  "pos " : Inport
  err : Inport  Port=2
  tr : Inport  Port=3
  Delay : Delay  DelayLength=1  InitialCondition=0
  Discrete Derivative : simulink/Discrete/Discrete Derivative  gainval=1.0  ICPrevScaledInput=0.0  OutMin=[]  OutMax=[]  OutDataType=fixdt(1, 16)  OutScaling=2^-10  DoSatur=off
  Discrete-Time Integrator : DiscreteIntegrator  ExternalReset=rising  SampleTime=-1  ICPrevOutput=DiscIntNeverNeededParam  ICPrevScaledInput=DiscIntNeverNeededParam
  Moving Average : dspstat3/Moving Average  Method=Sliding window  ForgettingFactorPort=off  SpecifyWindowLength=on  WindowLength=10  ForgettingFactor=0.9  SimulateUsing=Code generation
  Mux1 : Mux  Inputs=3
  Sum1 : Sum  Inputs=+|+
  Unary Minus : UnaryMinus
  x integration gain : Gain  Gain=slow.Kxi  Multiplication=Matrix(K*u)
  x matrix gain : Gain  Gain=slow.Kx  Multiplication=Matrix(K*u)
  V : Outport
  wires:
  x matrix gain/1 -> Sum1/1
  Mux1/1 -> x matrix gain/1  "x_vector"
  x integration gain/1 -> Sum1/2
  err/1 -> Discrete-Time Integrator/1, Mux1/2  "x_pos"
  Discrete-Time Integrator/1 -> x integration gain/1  "int_x"
  "pos "/1 -> Discrete Derivative/1
  Delay/1 -> Mux1/3
  Sum1/1 -> Delay/1, V/1
  tr/1 -> Discrete-Time Integrator/2  "x_pos"
  Discrete Derivative/1 -> Unary Minus/1
  Unary Minus/1 -> Moving Average/1
  Moving Average/1 -> Mux1/1

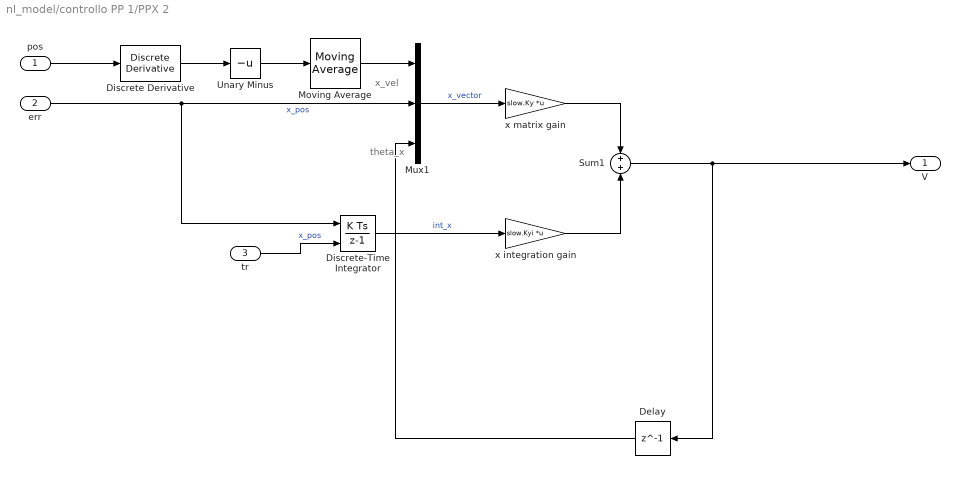
== system nl_model/controllo PP 1/PPX 2 ==
  note: theta_x
  note: x_vel
  "pos " : Inport
  err : Inport  Port=2
  tr : Inport  Port=3
  Delay : Delay  DelayLength=1  InitialCondition=0
  Discrete Derivative : simulink/Discrete/Discrete Derivative  gainval=1.0  ICPrevScaledInput=0.0  OutMin=[]  OutMax=[]  OutDataType=fixdt(1, 16)  OutScaling=2^-10  DoSatur=off
  Discrete-Time Integrator : DiscreteIntegrator  ExternalReset=rising  SampleTime=-1  ICPrevOutput=DiscIntNeverNeededParam  ICPrevScaledInput=DiscIntNeverNeededParam
  Moving Average : dspstat3/Moving Average  Method=Sliding window  ForgettingFactorPort=off  SpecifyWindowLength=on  WindowLength=10  ForgettingFactor=0.9  SimulateUsing=Code generation
  Mux1 : Mux  Inputs=3
  Sum1 : Sum  Inputs=+|+
  Unary Minus : UnaryMinus
  x integration gain : Gain  Gain=slow.Kyi  Multiplication=Matrix(K*u)
  x matrix gain : Gain  Gain=slow.Ky  Multiplication=Matrix(K*u)
  V : Outport
  wires:
  x matrix gain/1 -> Sum1/1
  Mux1/1 -> x matrix gain/1  "x_vector"
  x integration gain/1 -> Sum1/2
  err/1 -> Discrete-Time Integrator/1, Mux1/2  "x_pos"
  Discrete-Time Integrator/1 -> x integration gain/1  "int_x"
  "pos "/1 -> Discrete Derivative/1
  Delay/1 -> Mux1/3
  Sum1/1 -> Delay/1, V/1
  tr/1 -> Discrete-Time Integrator/2  "x_pos"
  Discrete Derivative/1 -> Unary Minus/1
  Unary Minus/1 -> Moving Average/1
  Moving Average/1 -> Mux1/1

== system nl_model/Subsystem1/Subsystem/BALL ==
  note: %input
      | geometrical constraints
      | %output
      | px ...............(m) spostamento X della palla
      | py ...............(m) spostamento Y della palla
      | pz ...............(m) spostamento Z della palla
  note: %ball
      | rho_ball=8000 ......................(kg/m^3) densita della sfera
      | R_ball=2 ...........................(cm) raggio della sfera
      | X_start=1 ..........................(cm) posizione X di partenza della palla
      | Y_start=1 ..........................(cm) posizione Y di partenza della palla
      | Z_start=0 ..........................(cm) posizione X di partenza della palla (Z=0 palla e piano in contatto)
  6-DOF Joint : sm_lib/Joints/6-DOF Joint  JointMode=Normal  SenseConstraintForce=off  SenseConstraintForceX=off  SenseConstraintForceY=off  SenseConstraintForceZ=off  SenseConstraintTorque=off  SenseConstraintTorqueX=off  SenseConstraintTorqueY=off  SenseConstraintTorqueZ=off  SenseTotalForce=off  SenseTotalForceX=off  SenseTotalForceY=off  SenseTotalForceZ=off  SenseTotalTorque=off  SenseTotalTorqueX=off  SenseTotalTorqueY=off  SenseTotalTorqueZ=off  CompositeWrenchDir=FollowerOnBase  CompositeWrenchFrame=BaseFrame  PxEquilibriumPosition=0  PxEquilibriumPositionUnits=m  PxSpringStiffness=0  PxSpringStiffnessUnits=N/m  PxDampingCoefficient=0  PxDampingCoefficientUnits=N/(m/s)  PxTorqueActuationMode=NoTorque  PxMotionActuationMode=ComputedMotion  PxSensePosition=on  PxSenseVelocity=off  PxSenseAcceleration=off  PxSenseTorqueForce=off  PxSenseLowerLimitTorqueForce=off  PxSenseUpperLimitTorqueForce=off  PxLowerLimitSpecify=off  PxLowerLimitBound=-1  PxLowerLimitBoundUnits=m  PxLowerLimitStiffness=1e6  PxLowerLimitStiffnessUnits=N/m  PxLowerLimitDamping=1e3  PxLowerLimitDampingUnits=N/(m/s)  PxLowerLimitTransitionRegionWidth=1e-4  PxLowerLimitTransitionRegionWidthUnits=m  PxUpperLimitSpecify=off  PxUpperLimitBound=1  PxUpperLimitBoundUnits=m  PxUpperLimitStiffness=1e6  PxUpperLimitStiffnessUnits=N/m  PxUpperLimitDamping=1e3  PxUpperLimitDampingUnits=N/(m/s)  PxUpperLimitTransitionRegionWidth=1e-4  PxUpperLimitTransitionRegionWidthUnits=m  PxPositionTargetSpecify=off  PxPositionTargetPriority=High  PxPositionTargetValue=0  PxPositionTargetValueUnits=m  PxVelocityTargetSpecify=off  PxVelocityTargetPriority=High  PxVelocityTargetValue=0  PxVelocityTargetValueUnits=m/s  PyEquilibriumPosition=0  PyEquilibriumPositionUnits=m  PySpringStiffness=0  PySpringStiffnessUnits=N/m  PyDampingCoefficient=0  PyDampingCoefficientUnits=N/(m/s)  PyTorqueActuationMode=NoTorque  PyMotionActuationMode=ComputedMotion  PySensePosition=on  PySenseVelocity=off  PySenseAcceleration=off  PySenseTorqueForce=off  PySenseLowerLimitTorqueForce=off  PySenseUpperLimitTorqueForce=off  PyLowerLimitSpecify=off  PyLowerLimitBound=-1  PyLowerLimitBoundUnits=m  PyLowerLimitStiffness=1e6  PyLowerLimitStiffnessUnits=N/m  PyLowerLimitDamping=1e3  PyLowerLimitDampingUnits=N/(m/s)  PyLowerLimitTransitionRegionWidth=1e-4  PyLowerLimitTransitionRegionWidthUnits=m  PyUpperLimitSpecify=off  PyUpperLimitBound=1  PyUpperLimitBoundUnits=m  PyUpperLimitStiffness=1e6  PyUpperLimitStiffnessUnits=N/m  PyUpperLimitDamping=1e3  PyUpperLimitDampingUnits=N/(m/s)  PyUpperLimitTransitionRegionWidth=1e-4  PyUpperLimitTransitionRegionWidthUnits=m  PyPositionTargetSpecify=off  PyPositionTargetPriority=High  PyPositionTargetValue=0  PyPositionTargetValueUnits=m  PyVelocityTargetSpecify=off  PyVelocityTargetPriority=High  PyVelocityTargetValue=0  PyVelocityTargetValueUnits=m/s  PzEquilibriumPosition=0  PzEquilibriumPositionUnits=m  PzSpringStiffness=0  PzSpringStiffnessUnits=N/m  PzDampingCoefficient=0  PzDampingCoefficientUnits=N/(m/s)  PzTorqueActuationMode=NoTorque  PzMotionActuationMode=ComputedMotion  PzSensePosition=on  PzSenseVelocity=off  PzSenseAcceleration=off  PzSenseTorqueForce=off  PzSenseLowerLimitTorqueForce=off  PzSenseUpperLimitTorqueForce=off  PzLowerLimitSpecify=off  PzLowerLimitBound=-1  PzLowerLimitBoundUnits=m  PzLowerLimitStiffness=1e6  PzLowerLimitStiffnessUnits=N/m  PzLowerLimitDamping=1e3  PzLowerLimitDampingUnits=N/(m/s)  PzLowerLimitTransitionRegionWidth=1e-4  PzLowerLimitTransitionRegionWidthUnits=m  PzUpperLimitSpecify=off  PzUpperLimitBound=1  PzUpperLimitBoundUnits=m  PzUpperLimitStiffness=1e6  PzUpperLimitStiffnessUnits=N/m  PzUpperLimitDamping=1e3  PzUpperLimitDampingUnits=N/(m/s)  PzUpperLimitTransitionRegionWidth=1e-4  PzUpperLimitTransitionRegionWidthUnits=m  PzPositionTargetSpecify=off  PzPositionTargetPriority=High  PzPositionTargetValue=0  PzPositionTargetValueUnits=m  PzVelocityTargetSpecify=off  PzVelocityTargetPriority=High  PzVelocityTargetValue=0  PzVelocityTargetValueUnits=m/s  SphDefPosRotationMethod=None  SphDefPosRotationAngleUnits=deg  SphDefPosRotationStandardAxis=+Z  SphDefPosRotationAngle=0.0  SphDefPosRotationArbitraryAxis=[0 0 1]  SphDefPosFollAlignAxisA=+X  SphDefPosBaseAlignAxisA=+Y  SphDefPosFollAlignAxisB=+Y  SphDefPosBaseAlignAxisB=+Z  SphDefPosRotationSequenceAxes=FollowerAxes  SphDefPosRotationSequence=XYX  SphDefPosRotationSequenceAngles=[0 0 0]  SphDefPosRotationSequenceAnglesUnits=deg  SphDefPosRotationMatrix=[1 0 0; 0 1 0; 0 0 1]  SphEqPosRotationMethod=None  SphEqPosRotationAngleUnits=deg  SphEqPosRotationStandardAxis=+Z  SphEqPosRotationAngle=0.0  SphEqPosRotationArbitraryAxis=[0 0 1]  SphEqPosFollAlignAxisA=+X  SphEqPosBaseAlignAxisA=+Y  SphEqPosFollAlignAxisB=+Y  SphEqPosBaseAlignAxisB=+Z  SphEqPosRotationSequenceAxes=FollowerAxes  SphEqPosRotationSequence=XYX  SphEqPosRotationSequenceAngles=[0 0 0]  SphEqPosRotationSequenceAnglesUnits=deg  SphEqPosRotationMatrix=[1 0 0; 0 1 0; 0 0 1]  SphSpringStiffness=0  SphSpringStiffnessUnits=N*m/deg  SphDampingCoefficient=0  SphDampingCoefficientUnits=N*m/(deg/s)  SphActuateTorqueX=off  SphActuateTorqueY=off  SphActuateTorqueZ=off  SphActuateTorque=off  SphTorqueActuationMode=NoTorque  SphMotionActuationMode=ComputedMotion  SphActuationFrame=BaseFrame  SphSensePosition=off  SphSenseVelocityX=off  SphSenseVelocityY=off  SphSenseVelocityZ=off  SphSenseVelocity=off  SphSenseAccelerationX=off  SphSenseAccelerationY=off  SphSenseAccelerationZ=off  SphSenseAcceleration=off  SphSenseTorqueX=off  SphSenseTorqueY=off  SphSenseTorqueZ=off  SphSenseTorqueForce=off  SphSenseLowerLimitTorqueMag=off  SphSenseUpperLimitTorqueMag=off  SphSensingFrame=BaseFrame  SphLowerLimitSpecify=off  SphLowerLimitBound=15  SphLowerLimitBoundUnits=deg  SphLowerLimitStiffness=1e4  SphLowerLimitStiffnessUnits=N*m/deg  SphLowerLimitDamping=10  SphLowerLimitDampingUnits=N*m/(deg/s)  SphLowerLimitTransitionRegionWidth=0.1  SphLowerLimitTransitionRegionWidthUnits=deg  SphUpperLimitSpecify=off  SphUpperLimitBound=45  SphUpperLimitBoundUnits=deg  SphUpperLimitStiffness=1e4  SphUpperLimitStiffnessUnits=N*m/deg  SphUpperLimitDamping=10  SphUpperLimitDampingUnits=N*m/(deg/s)  SphUpperLimitTransitionRegionWidth=0.1  SphUpperLimitTransitionRegionWidthUnits=deg  SphPositionTargetRotationMethod=None  SphPositionTargetRotationAngleUnits=deg  SphPositionTargetRotationStandardAxis=+Z  SphPositionTargetRotationAngle=0.0  SphPositionTargetRotationArbitraryAxis=[0 0 1]  SphPositionTargetFollAlignAxisA=+X  SphPositionTargetBaseAlignAxisA=+Y  SphPositionTargetFollAlignAxisB=+Y  SphPositionTargetBaseAlignAxisB=+Z  SphPositionTargetRotationSequenceAxes=FollowerAxes  SphPositionTargetRotationSequence=XYX  SphPositionTargetRotationSequenceAngles=[0 0 0]  SphPositionTargetRotationSequenceAnglesUnits=deg  SphPositionTargetRotationMatrix=[1 0 0; 0 1 0; 0 0 1]  SphPositionTargetSpecify=off  SphPositionTargetPriority=High  SphVelocityTargetValue=[0 0 0]  SphVelocityTargetValueUnits=deg/s  SphVelocityTargetSpecify=off  SphVelocityTargetPriority=High  SphVelocityTargetInFollowerFrame=on
  PS-Simulink Converter : nesl_utility/PS-Simulink Converter  PhysicalDomain=network_engine_domain  SubClassName=ps_output  LeftPortType=input  RightPortType=output  PseudoPeriodic=off  Frequencies=[]  Unit=inherit  AffineConversion=off
      settings: SourceProductBaseCode=PW,SS
  PS-Simulink Converter1 : nesl_utility/PS-Simulink Converter  PhysicalDomain=network_engine_domain  SubClassName=ps_output  LeftPortType=input  RightPortType=output  PseudoPeriodic=off  Frequencies=[]  Unit=inherit  AffineConversion=off
      settings: SourceProductBaseCode=PW,SS
  PS-Simulink Converter2 : nesl_utility/PS-Simulink Converter  PhysicalDomain=network_engine_domain  SubClassName=ps_output  LeftPortType=input  RightPortType=output  PseudoPeriodic=off  Frequencies=[]  Unit=inherit  AffineConversion=off
      settings: SourceProductBaseCode=PW,SS
  Spherical Solid : sm_lib/Body Elements/Spherical Solid  GraphicAmbientColor=[0.15 0.15 0.15 1.0]  BasedOnType=Density  CenterOfMass=[0 0 0]  CenterOfMassUnits=m  GraphicDiffuseColor=[0.0 0.8 0.2]  Density=rho_ball  DensityUnits=kg/m^3  DoExposeReferenceFrame=on  GraphicEmissiveColor=[0.0 0.0 0.0 1.0]  ExportEntireGeometry=on  SerializedExposedGeometries=<ExposedGeometries><ExposedGeometry><RawGeometryId>entire</RawGeometryId><ExposedGeometryId>G</ExposedGeometryId></ExposedGeometry></ExposedGeometries>  SerializedFrames=<Frames><Frame><Id>Frame1</Id><Value><Name>F1</Name><Origin><Source>ReferenceFrame</Source><FeatureName></FeatureName></Origin><PrimaryAxis><DefinedDirection>+Y</DefinedDirection><Source>ReferenceFrame</Source><SourceDirection>+Z</SourceDirection><FeatureName></FeatureName></PrimaryAxis><SecondaryAxis><DefinedDirection>-X</DefinedDirection><Source>ReferenceFrame</Source><SourceDirection>+X</SourceDirection><FeatureName></FeatureName></SecondaryAxis></Value></Frame></Frames>  MarkerShape=Sphere  MarkerSize=10  GraphicType=FromGeometry  InertiaType=CalculateFromGeometry  Mass=1  MassUnits=kg  MomentsOfInertia=[1 1 1]  MomentsOfInertiaUnits=kg*m^2  GraphicOpacity=1.0  ProductsOfInertia=[0 0 0]  ProductsOfInertiaUnits=kg*m^2  GraphicShininess=75  GraphicSpecularColor=[0.5 0.5 0.5 1.0]  SphereRadius=rb  SphereRadiusUnits=m  GraphicVisPropType=SimpleVisualProperties
  Conn1 : PMIOPort  Side=Right
  Conn2 : PMIOPort  Port=2  Side=Left
  Conn3 : PMIOPort  Port=3  Side=Left
  output : Outport
  output1 : Outport  Port=2
  output2 : Outport  Port=3
  wires:
  PS-Simulink Converter1/1 -> output1/1
  PS-Simulink Converter/1 -> output/1
  PS-Simulink Converter2/1 -> output2/1
  connections:
  6-DOF Joint/RConn4 -- PS-Simulink Converter2/LConn1
  6-DOF Joint/RConn2 -- PS-Simulink Converter/LConn1
  Spherical Solid/RConn1 -- Conn1/RConn1
  6-DOF Joint/RConn1 -- Spherical Solid/LConn1
  6-DOF Joint/LConn1 -- Conn3/RConn1
  6-DOF Joint/RConn3 -- PS-Simulink Converter1/LConn1
  Conn2/RConn1 -- Spherical Solid/LConn2
